simulink model "quadcopter_model_c_NewtonEuler"  (Simulink 8.7)
settings: Solver=VariableStepAuto  StartTime=0.0  StopTime=100  RelTol=1e-3
undefined symbols (not defined in the file): A, g, I, m
libraries: aerolibutil x1
settings Model: Creator=Daniel  LastModifiedBy=mgreiff
settings DataIOCC: SaveFormat=Dataset
settings DebuggingCC: UnderspecifiedInitializationDetection=Simplified  MergeDetectMultiDrivingBlocksExec=error  AllowSymbolicDim=off
settings HardwareCC: ProdBitPerPointer=64  ProdLargestAtomicFloat=Float  ProdIntDivRoundTo=Zero  ProdEndianess=LittleEndian  ProdWordSize=64  ProdHWDeviceType=Intel->x86-64 (Windows64)
settings GRTTargetCC: GeneratePreprocessorConditionals=Use local settings
settings ConfigComp: CovModelRefEnable=off

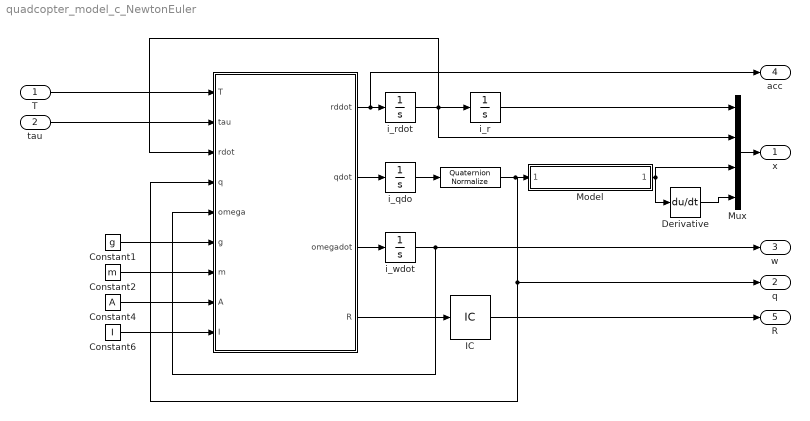
== system quadcopter_model_c_NewtonEuler ==
  T : Inport  PortDimensions=1
  tau : Inport  Port=2  PortDimensions=3
  " " : MATLAB Function  TreatAsAtomicUnit=on
  "  " : aerolibutil/Quaternion Normalize
  Constant1 : Constant  Value=g
  Constant2 : Constant  Value=m
  Constant4 : Constant  Value=A
  Constant6 : Constant  Value=I
  Derivative : Derivative
  IC : InitialCondition  Value=eye(3)
  Model : ModelReference  ModelNameDialog=quaternion2euler.mdl  SimulationMode=Normal  ModelReferenceVersion=1.92
  Mux : Mux
  i_qdo : Integrator  InitialCondition=[1; 0; 0; 0]
  i_r : Integrator  InitialCondition=[0 0 0]'
  i_rdot : Integrator  InitialCondition=[0; 0; 0]
  i_wdot : Integrator  InitialCondition=[0; 0; 0]
  x : Outport  PortDimensions=12
  q : Outport  Port=2  PortDimensions=4
  w : Outport  Port=3  PortDimensions=3
  acc : Outport  Port=4  PortDimensions=3
  R : Outport  Port=5
  wires:
  " "/2(qdot) -> i_qdo/1
  " "/1(rddot) -> acc/1, i_rdot/1
  i_r/1 -> Mux/1
  T/1 -> " "/1(T)
  i_rdot/1 -> Mux/2, i_r/1, " "/3(rdot)
  tau/1 -> " "/2(tau)
  " "/3(omegadot) -> i_wdot/1
  Constant1/1 -> " "/6(g)
  Constant2/1 -> " "/7(m)
  Constant4/1 -> " "/8(A)
  Constant6/1 -> " "/9(I)
  i_wdot/1 -> w/1, " "/5(omega)
  i_qdo/1 -> "  "/1
  " "/4(R) -> IC/1
  "  "/1 -> " "/4(q), q/1, Model/1
  Model/1 -> Mux/3, Derivative/1
  Derivative/1 -> Mux/4
  Mux/1 -> x/1
  IC/1 -> R/1

== matlab function   ==
  data: T input double; tau input double; rddot output double; rdot input double; q input double; omega input double; qdot output double; g input double; m input double; A input double; I input double; omegadot output double; R output double
function [ rddot,qdot,omegadot, R] = quad_acceleration(T, tau, rdot, q, omega, g, m, A, I)

    qw = q(1); qx = q(2); qy = q(3); qz = q(4); qv = q(2:4);
    omegaw = 0; omegav = omega;
    
%     % Gravity acceleration
%     Ga = -g * [0; 0; 1];
% 
%     % TODO write rotation
%     angM = [2*(qx*qz + qw*qy);
%             2*(qy*qz - qw*qx);
%             qw.^2 - qx.^2 - qy.^2 + qz.^2];
% 
%     Ta = (T/m) .* angM;
% 
%     % Drag
%     Aa = -1/m * diag(A) * rdot;
%     rddot = Ga + Ta + Aa;
%     
%     % Define the C-matrix as (19)
%     J = diag(I);
%     %qdot = -0.5.*[qv'*omegav; qw.*omegav + qv.*omegaw + cross(qv, omegav)];
%     qdot = 0.5.*[omegav'*qv; omegav.*qw + omegaw.*qv + cross(omegav, qv)];
%     omegadot = J\(tau - cross(omegav, J*omegav));
% 
%     % TODO write out R for visualization if need be
%     R = eye(3);
    % Gravity acceleration
    Ga = -g * [0; 0; 1];

    % TODO write rotation
    angM = [2*(qx*qz + qw*qy);
            2*(qy*qz - qw*qx);
            qw.^2 - qx.^2 - qy.^2 + qz.^2];

    Ta = (T/m) .* angM;

    % Drag
    Aa = -1/m * diag(A) * rdot;
    rddot = Ga + Ta + Aa;
    
    % Define the C-matrix as (19)
    J = diag(I);
    qcross = [0, -qz, qy; qz, 0, -qx; -qy, qx, 0];
    %qdot = -0.5.*[qv'*omegav; qw.*omegav + qv.*omegaw + cross(qv, omegav)];
    qdot = 0.5.*(eye(4)*qw  + [0, -qv';qv, qcross])*[0; omegav];
    omegadot = J\(tau - cross(omegav, J*omegav));

    % TODO write out R for visualization if need be
    R = [qw^2+qx^2+qy^2+qz^2, 2*(qx*qy-qw*qz)    , 2*(qx*qz+qw*qy);
         2*(qx*qy+qw*qz)    , qw^2-qx^2+qy^2-qz^2, 2*(qy*qz-qw*qx);
         2*(qx*qz-qw*qy)    , 2*(qy*qz+qw*qx)    , qw^2-qx^2-qy^2+qz^2];
end
